simulink model "exampleSaturationValueWater"  (Simulink 7.6)
settings: Solver=ode45  StartTime=0.0  StopTime=10.0  RelTol=1e-3
libraries: carnot x3
settings Model: Creator=drhf  LastModifiedBy=drhf

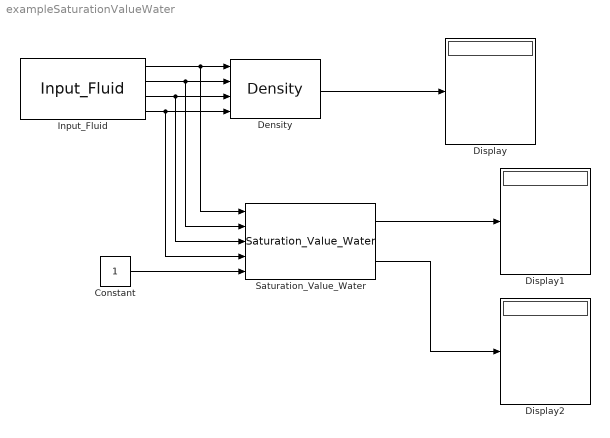
== system exampleSaturationValueWater ==
  Constant : Constant
  Density : carnot/Basic/Material_Properties/Density  SystemSampleTime=-1
  Display : Display
  Display1 : Display
  Display2 : Display
  Input_Fluid : carnot/Basic/Material_Properties/Input_Fluid  SystemSampleTime=-1  fluid=water  T=10:20:90  p=1e5  x=0
  Saturation_Value_Water : carnot/Basic/Material_Properties/Saturation_Value_Water  SystemSampleTime=-1
  wires:
  Input_Fluid/1 -> Density/1, Saturation_Value_Water/1
  Input_Fluid/2 -> Density/2, Saturation_Value_Water/2
  Input_Fluid/3 -> Density/3, Saturation_Value_Water/3
  Input_Fluid/4 -> Density/4, Saturation_Value_Water/4
  Density/1 -> Display/1
  Constant/1 -> Saturation_Value_Water/5
  Saturation_Value_Water/1 -> Display1/1
  Saturation_Value_Water/2 -> Display2/1
